simulink library "inp"  (R2021b)
settings: Solver=VariableStepAuto  StartTime=0.0  StopTime=10.0  RelTol=1e-3
undefined symbols (not defined in the file): C_TASK_5MS_S, FALSE, KINP_AcoreReadyToSlp_flg_ovrdflg, KINP_AcoreReadyToSlp_flg_ovrdval, KINP_AllowMovThd_OTA_enum_ovrdflg, KINP_AllowMovThd_OTA_enum_ovrdval, KINP_APSAngleTarget_Deg_ovrdflg, KINP_APSAngleTarget_Deg_ovrdval, KINP_APSDecReq_mps2_ovrdflg, KINP_APSDecReq_mps2_ovrdval, KINP_APSDecReqA_flg_ovrdflg, KINP_APSDecReqA_flg_ovrdval, KINP_APSDFLL_cm_ovrdflg, KINP_APSDFLL_cm_ovrdval, KINP_APSDFLR_cm_ovrdflg, KINP_APSDFLR_cm_ovrdval, KINP_APSDRLL_cm_ovrdflg, KINP_APSDRLL_cm_ovrdval, KINP_APSDRLR_cm_ovrdflg, KINP_APSDRLR_cm_ovrdval, KINP_APSExitCondition_enum_ovrdflg, KINP_APSExitCondition_enum_ovrdval, KINP_APSHWVer_enum_ovrdflg, KINP_APSHWVer_enum_ovrdval, KINP_APSProgressPCT_pct_ovrdflg, KINP_APSProgressPCT_pct_ovrdval, KINP_APSPwrReq_enum_ovrdflg, KINP_APSPwrReq_enum_ovrdval, KINP_APSReq_enum_ovrdflg, KINP_APSReq_enum_ovrdval, KINP_APSRQDisplay_enum_ovrdflg, KINP_APSRQDisplay_enum_ovrdval, KINP_APSRqEPASCtrl_flg_ovrdflg, KINP_APSRqEPASCtrl_flg_ovrdval, KINP_APSShiftPosnReq_enum_ovrdval, KINP_APSShiftPosnReq_enum_ovrflg, KINP_APSSpeedCMD_kph_ovrdval, KINP_APSSpeedCMD_kph_ovrflg, KINP_APSStaSystem_enum_ovrdflg, KINP_APSStaSystem_enum_ovrdval, KINP_APSSWVer_enum_ovrdflg, KINP_APSSWVer_enum_ovrdval, KINP_APSVMCReqA_flg_ovrdval, KINP_APSVMCReqA_flg_ovrflg, KINP_APSVRqEPASCtrl_flg_ovrdflg, KINP_APSVRqEPASCtrl_flg_ovrdval, KINP_AuxBattVolmV_mV_ovrdflg, KINP_AuxBattVolmV_mV_ovrdval, KINP_CAASSta_enum_ovrdflg, KINP_CAASSta_enum_ovrdval, KINP_CAASVMCReqA_flg_ovrdval, KINP_CAASVMCReqA_flg_ovrflg, KINP_CAN1BusOff_flg_ovrdflg, KINP_CAN1BusOff_flg_ovrdval, KINP_CAN2BusOff_flg_ovrdflg, KINP_CAN2BusOff_flg_ovrdval, KINP_CAN3BusOff_flg_ovrdflg, KINP_CAN3BusOff_flg_ovrdval, KINP_CAN4BusOff_flg_ovrdflg, KINP_CAN4BusOff_flg_ovrdval ... (+152)
libraries: FVT_lib x1037, hcu_lib x1
(part 13 of 34)

== system inp/INP/CAN1/SignalCheck/EPS1 ==
  BHAL_outputs : Inport
  inp_CanValid_bus : Inport  Port=2
  DriIntend : FVT_lib/inp/can_signal_template  SystemSampleTime=-1  VariantActivationTime=update diagram  Latency=0  AutoFrameSizeCalculation=off
      link override defval: Value=KINP_DriIntend_enum_defval
      link override ovrdflg: Value=KINP_DriIntend_enum_ovrdflg
      link override ovrdval: Value=KINP_DriIntend_enum_ovrdval
  EPS1CSErr : FVT_lib/inp/can_signal_template  SystemSampleTime=-1  VariantActivationTime=update diagram  Latency=0  AutoFrameSizeCalculation=off
      link override defval: Value=KINP_EPS1CSErr_flg_defval
      link override ovrdflg: Value=KINP_EPS1CSErr_flg_ovrdflg
      link override ovrdval: Value=KINP_EPS1CSErr_flg_ovrdval
  EPS1RCErr : FVT_lib/inp/can_signal_template  SystemSampleTime=-1  VariantActivationTime=update diagram  Latency=0  AutoFrameSizeCalculation=off
      link override defval: Value=KINP_EPS1RCErr_flg_defval
      link override ovrdflg: Value=KINP_EPS1RCErr_flg_ovrdflg
      link override ovrdval: Value=KINP_EPS1RCErr_flg_ovrdval
  EPSAOIControl : FVT_lib/inp/can_signal_template  SystemSampleTime=-1  VariantActivationTime=update diagram  Latency=0  AutoFrameSizeCalculation=off
      link override defval: Value=KINP_EPSAOIControl_enum_defval
      link override ovrdflg: Value=KINP_EPSAOIControl_enum_ovrdflg
      link override ovrdval: Value=KINP_EPSAOIControl_enum_ovrdval
  EPSRC : FVT_lib/inp/can_signal_template  SystemSampleTime=-1  VariantActivationTime=update diagram  Latency=0  AutoFrameSizeCalculation=off
      link override defval: Value=KINP_EPSRC_enum_defval
      link override ovrdflg: Value=KINP_EPSRC_enum_ovrdflg
      link override ovrdval: Value=KINP_EPSRC_enum_ovrdval
  EPSTOIActivation : FVT_lib/inp/can_signal_template  SystemSampleTime=-1  VariantActivationTime=update diagram  Latency=0  AutoFrameSizeCalculation=off
      link override defval: Value=KINP_EPSTOIActivation_flg_defval
      link override ovrdflg: Value=KINP_EPSTOIActivation_flg_ovrdflg
      link override ovrdval: Value=KINP_EPSTOIActivation_flg_ovrdval
  EPSTOIFault : FVT_lib/inp/can_signal_template  SystemSampleTime=-1  VariantActivationTime=update diagram  Latency=0  AutoFrameSizeCalculation=off
      link override defval: Value=KINP_EPSTOIFault_flg_defval
      link override ovrdflg: Value=KINP_EPSTOIFault_flg_ovrdflg
      link override ovrdval: Value=KINP_EPSTOIFault_flg_ovrdval
  EPSTOIUnavailable : FVT_lib/inp/can_signal_template  SystemSampleTime=-1  VariantActivationTime=update diagram  Latency=0  AutoFrameSizeCalculation=off
      link override defval: Value=KINP_EPSTOIUnavailable_flg_defval
      link override ovrdflg: Value=KINP_EPSTOIUnavailable_flg_ovrdflg
      link override ovrdval: Value=KINP_EPSTOIUnavailable_flg_ovrdval
  EpasFailed : FVT_lib/inp/can_signal_template  SystemSampleTime=-1  VariantActivationTime=update diagram  Latency=0  AutoFrameSizeCalculation=off
      link override defval: Value=KINP_EpasFailed_enum_defval
      link override ovrdflg: Value=KINP_EpasFailed_enum_ovrdflg
      link override ovrdval: Value=KINP_EpasFailed_enum_ovrdval
  SASAngle : FVT_lib/inp/can_signal_template  SystemSampleTime=-1  VariantActivationTime=update diagram  Latency=0  AutoFrameSizeCalculation=off
      link override defval: Value=KINP_SASAngle_Deg_defval
      link override ovrdflg: Value=KINP_SASAngle_Deg_ovrdflg
      link override ovrdval: Value=KINP_SASAngle_Deg_ovrdval
  SASCAL : FVT_lib/inp/can_signal_template  SystemSampleTime=-1  VariantActivationTime=update diagram  Latency=0  AutoFrameSizeCalculation=off
      link override defval: Value=KINP_SASCAL_flg_defval
      link override ovrdflg: Value=KINP_SASCAL_flg_ovrdflg
      link override ovrdval: Value=KINP_SASCAL_flg_ovrdval
  SASSpeed : FVT_lib/inp/can_signal_template  SystemSampleTime=-1  VariantActivationTime=update diagram  Latency=0  AutoFrameSizeCalculation=off
      link override defval: Value=KINP_SASSpeed_degps_defval
      link override ovrdflg: Value=KINP_SASSpeed_degps_ovrdflg
      link override ovrdval: Value=KINP_SASSpeed_degps_ovrdval
  SASSpeedValid : FVT_lib/inp/can_signal_template  SystemSampleTime=-1  VariantActivationTime=update diagram  Latency=0  AutoFrameSizeCalculation=off
      link override defval: Value=KINP_SASSpeedValid_flg_defval
      link override ovrdflg: Value=KINP_SASSpeedValid_flg_ovrdflg
      link override ovrdval: Value=KINP_SASSpeedValid_flg_ovrdval
  SASV : FVT_lib/inp/can_signal_template  SystemSampleTime=-1  VariantActivationTime=update diagram  Latency=0  AutoFrameSizeCalculation=off
      link override defval: Value=KINP_SASV_flg_defval
      link override ovrdflg: Value=KINP_SASV_flg_ovrdflg
      link override ovrdval: Value=KINP_SASV_flg_ovrdval
  Terminator_{1..14} (14 alike) : Terminator
  True_VHAL_DriIntend_enum : Constant  Value=TRUE  OutDataTypeStr=boolean
  True_VHAL_EPS1CSErr_flg : Constant  Value=TRUE  OutDataTypeStr=boolean
  True_VHAL_EPS1RCErr_flg : Constant  Value=TRUE  OutDataTypeStr=boolean
  True_VHAL_EPSAOIControl_enum : Constant  Value=TRUE  OutDataTypeStr=boolean
  True_VHAL_EPSRC_enum : Constant  Value=TRUE  OutDataTypeStr=boolean
  True_VHAL_EPSTOIActivation_flg : Constant  Value=TRUE  OutDataTypeStr=boolean
  True_VHAL_EPSTOIFault_flg : Constant  Value=TRUE  OutDataTypeStr=boolean
  True_VHAL_EPSTOIUnavailable_flg : Constant  Value=TRUE  OutDataTypeStr=boolean
  True_VHAL_EpasFailed_enum : Constant  Value=TRUE  OutDataTypeStr=boolean
  True_VHAL_SASAngle_Deg : Constant  Value=TRUE  OutDataTypeStr=boolean
  True_VHAL_SASCAL_flg : Constant  Value=TRUE  OutDataTypeStr=boolean
  True_VHAL_SASSpeedValid_flg : Constant  Value=TRUE  OutDataTypeStr=boolean
  True_VHAL_SASSpeed_degps : Constant  Value=TRUE  OutDataTypeStr=boolean
  True_VHAL_SASV_flg : Constant  Value=TRUE  OutDataTypeStr=boolean
  slr1_{1..14} (14 alike) : BusSelector  OutputSignals=VINP_CANMsgValidEPS1_flg
  slr_VHAL_DriIntend_enum : BusSelector  OutputSignals=VHAL_DriIntend_enum
  slr_VHAL_EPS1CSErr_flg : BusSelector  OutputSignals=VHAL_EPS1CSErr_flg
  slr_VHAL_EPS1RCErr_flg : BusSelector  OutputSignals=VHAL_EPS1RCErr_flg
  slr_VHAL_EPSAOIControl_enum : BusSelector  OutputSignals=VHAL_EPSAOIControl_enum
  slr_VHAL_EPSRC_enum : BusSelector  OutputSignals=VHAL_EPSRC_enum
  slr_VHAL_EPSTOIActivation_flg : BusSelector  OutputSignals=VHAL_EPSTOIActivation_flg
  slr_VHAL_EPSTOIFault_flg : BusSelector  OutputSignals=VHAL_EPSTOIFault_flg
  slr_VHAL_EPSTOIUnavailable_flg : BusSelector  OutputSignals=VHAL_EPSTOIUnavailable_flg
  slr_VHAL_EpasFailed_enum : BusSelector  OutputSignals=VHAL_EpasFailed_enum
  slr_VHAL_SASAngle_Deg : BusSelector  OutputSignals=VHAL_SASAngle_Deg
  slr_VHAL_SASCAL_flg : BusSelector  OutputSignals=VHAL_SASCAL_flg
  slr_VHAL_SASSpeedValid_flg : BusSelector  OutputSignals=VHAL_SASSpeedValid_flg
  slr_VHAL_SASSpeed_degps : BusSelector  OutputSignals=VHAL_SASSpeed_degps
  slr_VHAL_SASV_flg : BusSelector  OutputSignals=VHAL_SASV_flg
  VINP_EPS1CSErr_flg : Outport
  VINP_EPS1RCErr_flg : Outport  Port=2
  VINP_DriIntend_enum : Outport  Port=3
  VINP_EPSAOIControl_enum : Outport  Port=4
  VINP_EPSRC_enum : Outport  Port=5
  VINP_EPSTOIActivation_flg : Outport  Port=6
  VINP_EPSTOIFault_flg : Outport  Port=7
  VINP_EPSTOIUnavailable_flg : Outport  Port=8
  VINP_EpasFailed_enum : Outport  Port=9
  VINP_SASAngle_Deg : Outport  Port=10
  VINP_SASCAL_flg : Outport  Port=11
  VINP_SASSpeed_degps : Outport  Port=12
  VINP_SASSpeedValid_flg : Outport  Port=13
  VINP_SASV_flg : Outport  Port=14
  wires:
  BHAL_outputs/1 -> [BHAL_outputs]
  inp_CanValid_bus/1 -> [inp_CanValid_bus]
  [BHAL_outputs] -> slr_VHAL_EPS1CSErr_flg/1
  slr_VHAL_EPS1CSErr_flg/1 -> EPS1CSErr/1  "<VHAL_EPS1CSErr_flg>"
  True_VHAL_EPS1CSErr_flg/1 -> EPS1CSErr/2
  [inp_CanValid_bus] -> slr1_1/1
  slr1_1/1 -> EPS1CSErr/3  "<VINP_CANMsgValidEPS1_flg>"
  EPS1CSErr/1 -> VINP_EPS1CSErr_flg/1  "VINP_EPS1CSErr_flg"
  EPS1CSErr/2 -> Terminator_1/1
  [BHAL_outputs] -> slr_VHAL_EPS1RCErr_flg/1
  slr_VHAL_EPS1RCErr_flg/1 -> EPS1RCErr/1  "<VHAL_EPS1RCErr_flg>"
  True_VHAL_EPS1RCErr_flg/1 -> EPS1RCErr/2
  [inp_CanValid_bus] -> slr1_2/1
  slr1_2/1 -> EPS1RCErr/3  "<VINP_CANMsgValidEPS1_flg>"
  EPS1RCErr/1 -> VINP_EPS1RCErr_flg/1  "VINP_EPS1RCErr_flg"
  EPS1RCErr/2 -> Terminator_2/1
  [BHAL_outputs] -> slr_VHAL_DriIntend_enum/1
  slr_VHAL_DriIntend_enum/1 -> DriIntend/1  "<VHAL_DriIntend_enum>"
  True_VHAL_DriIntend_enum/1 -> DriIntend/2
  [inp_CanValid_bus] -> slr1_3/1
  slr1_3/1 -> DriIntend/3  "<VINP_CANMsgValidEPS1_flg>"
  DriIntend/1 -> VINP_DriIntend_enum/1  "VINP_DriIntend_enum"
  DriIntend/2 -> Terminator_3/1
  [BHAL_outputs] -> slr_VHAL_EPSAOIControl_enum/1
  slr_VHAL_EPSAOIControl_enum/1 -> EPSAOIControl/1  "<VHAL_EPSAOIControl_enum>"
  True_VHAL_EPSAOIControl_enum/1 -> EPSAOIControl/2
  [inp_CanValid_bus] -> slr1_4/1
  slr1_4/1 -> EPSAOIControl/3  "<VINP_CANMsgValidEPS1_flg>"
  EPSAOIControl/1 -> VINP_EPSAOIControl_enum/1  "VINP_EPSAOIControl_enum"
  EPSAOIControl/2 -> Terminator_4/1
  [BHAL_outputs] -> slr_VHAL_EPSRC_enum/1
  slr_VHAL_EPSRC_enum/1 -> EPSRC/1  "<VHAL_EPSRC_enum>"
  True_VHAL_EPSRC_enum/1 -> EPSRC/2
  [inp_CanValid_bus] -> slr1_5/1
  slr1_5/1 -> EPSRC/3  "<VINP_CANMsgValidEPS1_flg>"
  EPSRC/1 -> VINP_EPSRC_enum/1  "VINP_EPSRC_enum"
  EPSRC/2 -> Terminator_5/1
  [BHAL_outputs] -> slr_VHAL_EPSTOIActivation_flg/1
  slr_VHAL_EPSTOIActivation_flg/1 -> EPSTOIActivation/1  "<VHAL_EPSTOIActivation_flg>"
  True_VHAL_EPSTOIActivation_flg/1 -> EPSTOIActivation/2
  [inp_CanValid_bus] -> slr1_6/1
  slr1_6/1 -> EPSTOIActivation/3  "<VINP_CANMsgValidEPS1_flg>"
  EPSTOIActivation/1 -> VINP_EPSTOIActivation_flg/1  "VINP_EPSTOIActivation_flg"
  EPSTOIActivation/2 -> Terminator_6/1
  [BHAL_outputs] -> slr_VHAL_EPSTOIFault_flg/1
  slr_VHAL_EPSTOIFault_flg/1 -> EPSTOIFault/1  "<VHAL_EPSTOIFault_flg>"
  True_VHAL_EPSTOIFault_flg/1 -> EPSTOIFault/2
  [inp_CanValid_bus] -> slr1_7/1
  slr1_7/1 -> EPSTOIFault/3  "<VINP_CANMsgValidEPS1_flg>"
  EPSTOIFault/1 -> VINP_EPSTOIFault_flg/1  "VINP_EPSTOIFault_flg"
  EPSTOIFault/2 -> Terminator_7/1
  [BHAL_outputs] -> slr_VHAL_EPSTOIUnavailable_flg/1
  slr_VHAL_EPSTOIUnavailable_flg/1 -> EPSTOIUnavailable/1  "<VHAL_EPSTOIUnavailable_flg>"
  True_VHAL_EPSTOIUnavailable_flg/1 -> EPSTOIUnavailable/2
  [inp_CanValid_bus] -> slr1_8/1
  slr1_8/1 -> EPSTOIUnavailable/3  "<VINP_CANMsgValidEPS1_flg>"
  EPSTOIUnavailable/1 -> VINP_EPSTOIUnavailable_flg/1  "VINP_EPSTOIUnavailable_flg"
  EPSTOIUnavailable/2 -> Terminator_8/1
  [BHAL_outputs] -> slr_VHAL_EpasFailed_enum/1
  slr_VHAL_EpasFailed_enum/1 -> EpasFailed/1  "<VHAL_EpasFailed_enum>"
  True_VHAL_EpasFailed_enum/1 -> EpasFailed/2
  [inp_CanValid_bus] -> slr1_9/1
  slr1_9/1 -> EpasFailed/3  "<VINP_CANMsgValidEPS1_flg>"
  EpasFailed/1 -> VINP_EpasFailed_enum/1  "VINP_EpasFailed_enum"
  EpasFailed/2 -> Terminator_9/1
  [BHAL_outputs] -> slr_VHAL_SASAngle_Deg/1
  slr_VHAL_SASAngle_Deg/1 -> SASAngle/1  "<VHAL_SASAngle_Deg>"
  True_VHAL_SASAngle_Deg/1 -> SASAngle/2
  [inp_CanValid_bus] -> slr1_10/1
  slr1_10/1 -> SASAngle/3  "<VINP_CANMsgValidEPS1_flg>"
  SASAngle/1 -> VINP_SASAngle_Deg/1  "VINP_SASAngle_Deg"
  SASAngle/2 -> Terminator_10/1
  [BHAL_outputs] -> slr_VHAL_SASCAL_flg/1
  slr_VHAL_SASCAL_flg/1 -> SASCAL/1  "<VHAL_SASCAL_flg>"
  True_VHAL_SASCAL_flg/1 -> SASCAL/2
  [inp_CanValid_bus] -> slr1_11/1
  slr1_11/1 -> SASCAL/3  "<VINP_CANMsgValidEPS1_flg>"
  SASCAL/1 -> VINP_SASCAL_flg/1  "VINP_SASCAL_flg"
  SASCAL/2 -> Terminator_11/1
  [BHAL_outputs] -> slr_VHAL_SASSpeed_degps/1
  slr_VHAL_SASSpeed_degps/1 -> SASSpeed/1  "<VHAL_SASSpeed_degps>"
  True_VHAL_SASSpeed_degps/1 -> SASSpeed/2
  [inp_CanValid_bus] -> slr1_12/1
  slr1_12/1 -> SASSpeed/3  "<VINP_CANMsgValidEPS1_flg>"
  SASSpeed/1 -> VINP_SASSpeed_degps/1  "VINP_SASSpeed_degps"
  SASSpeed/2 -> Terminator_12/1
  [BHAL_outputs] -> slr_VHAL_SASSpeedValid_flg/1
  slr_VHAL_SASSpeedValid_flg/1 -> SASSpeedValid/1  "<VHAL_SASSpeedValid_flg>"
  True_VHAL_SASSpeedValid_flg/1 -> SASSpeedValid/2
  [inp_CanValid_bus] -> slr1_13/1
  slr1_13/1 -> SASSpeedValid/3  "<VINP_CANMsgValidEPS1_flg>"
  SASSpeedValid/1 -> VINP_SASSpeedValid_flg/1  "VINP_SASSpeedValid_flg"
  SASSpeedValid/2 -> Terminator_13/1
  [BHAL_outputs] -> slr_VHAL_SASV_flg/1
  slr_VHAL_SASV_flg/1 -> SASV/1  "<VHAL_SASV_flg>"
  True_VHAL_SASV_flg/1 -> SASV/2
  [inp_CanValid_bus] -> slr1_14/1
  slr1_14/1 -> SASV/3  "<VINP_CANMsgValidEPS1_flg>"
  SASV/1 -> VINP_SASV_flg/1  "VINP_SASV_flg"
  SASV/2 -> Terminator_14/1
